simulink model "Motor_ctrl_INST"  (R2025b)
settings: Solver=ode15s  StartTime=0.0  StopTime=1  FixedStep=Ts/10  MaxStep=Tstep  RelTol=1e-3  AbsTol=1e-3  EnableMultiTasking=on
InitFcn:
  | if ~exist('flagwp')
  |     tic
  |     init_sim
  | end
  | mex Motor_ctrl.c User_functions/Src/*.c
StopFcn:
  | if ~exist('flagwp')
  |   elapsed_time=toc
  | end
values from neighbouring files (symbols this model uses):
  accel = 5000    [init_sim.m]
  Bm = 0    [init_sim.m]
  Clarke_inv = [1 0;-0.5 sqrt(3)/2;-0.5 -sqrt(3)/2]    [init_sim.m]
  Ctrl_strategy = 1    [init_sim.m]
  Ctrl_type = 3    [init_sim.m]
  dem = 1    [init_sim.m]
  dT = motorModel.SyreDrive.Converter.dT * 1e-6    [init_sim.m]
  expC = motorModel.IronPMLossMap_dq.expC    [init_sim.m]
  expH = motorModel.IronPMLossMap_dq.expH    [init_sim.m]
  expPM = motorModel.IronPMLossMap_dq.expPM    [init_sim.m]
  Fd0 = interp2(motorModel.FluxMap_dq.Id,motorModel.FluxMap_dq.Iq,motorModel.FluxMap_dq.Fd,0,0)    [init_sim.m]
  Fm = interp2(Idd,Iqq,Fdd,0,0)    [init_sim.m]
  HS_ctrl = 1    [init_sim.m]
  Id_dqt = interpn(motorModel.FluxMapInv_dqt.dataF.Fd,motorModel.FluxMapInv_dqt.dataF.Fq,motorModel.FluxMapInv_dqt.dataF.th,motorModel.FluxMapInv_dqt.dataF.Id,Fd_dqt,Fq_dqt,th_dqt,'cubic')    [init_sim.m]
  Id_fe = motorModel.IronPMLossMap_dq.Id    [init_sim.m]
  InitIntg_d = Fm*cos(th0)    [init_sim.m]
  InitIntg_q = Fm*sin(th0)    [init_sim.m]
  inj_waveform = 1    [init_sim.m]
  Iq_dqt = interpn(motorModel.FluxMapInv_dqt.dataF.Fd,motorModel.FluxMapInv_dqt.dataF.Fq,motorModel.FluxMapInv_dqt.dataF.th,motorModel.FluxMapInv_dqt.dataF.Iq,Fd_dqt,Fq_dqt,th_dqt,'cubic')    [init_sim.m]
  Iq_fe = motorModel.IronPMLossMap_dq.Iq    [init_sim.m]
  IronLoss = 1    [init_sim.m]
  J = motorModel.data.J    [init_sim.m]
  n0 = motorModel.IronPMLossMap_dq.n0    [init_sim.m]
  p = motorModel.data.p    [init_sim.m]
  Pfe_c = motorModel.IronPMLossMap_dq.Pfes_c + motorModel.IronPMLossMap_dq.Pfer_c    [init_sim.m]
  Pfe_h = motorModel.IronPMLossMap_dq.Pfes_h + motorModel.IronPMLossMap_dq.Pfer_h    [init_sim.m]
  Ppm = motorModel.IronPMLossMap_dq.Ppm    [init_sim.m]
  Quad_Maps = 2    [init_sim.m]
  SS_on = 1    [init_sim.m]
  T_dqt = interpn(motorModel.FluxMapInv_dqt.dataF.Fd,motorModel.FluxMapInv_dqt.dataF.Fq,motorModel.FluxMapInv_dqt.dataF.th,motorModel.FluxMapInv_dqt.dataF.T,Fd_dqt,Fq_dqt,th_dqt,'cubic')    [init_sim.m]
  Tf = 0    [init_sim.m]
  th0 = 0    [init_sim.m]
  th_max = max(motorModel.FluxMapInv_dqt.dataF.th,[],'all')    [init_sim.m]
  th_min = min(motorModel.FluxMapInv_dqt.dataF.th,[],'all')    [init_sim.m]
  Ts = 1/motorModel.SyreDrive.Converter.fPWM    [init_sim.m]
  Tv = 0    [init_sim.m]
  VDC = motorModel.data.Vdc    [init_sim.m]
undefined symbols (not defined in the file or in its folder): ACloss, eMotor, fD_pu_norm, fD_vct_max, fD_vct_ref, fQ_pu_norm, fQ_vct_max, fQ_vct_ref, iD_pu_norm, idRef, interpn, iQ_pu_norm, iqRef, J_rot, magnitude, motorModelType, nRef, sigbuilder_block, T0
libraries: nesl_utility x43, fl_lib x41, ee_lib x8, simulink x8, eeTransforms x1
(part 4 of 4)

== system Motor_ctrl_INST/Power block - Inverter + Motor/Noncircuital/FM/Motor Model/Inverse Flux Maps/2D LUT/dq Model/SyR/Fdq -> idq ==
  Fdq : Inport
  1-D Lookup Table : Lookup_n-D  NumberOfTableDimensions=1  BreakpointsForDimension1=fD_vct_ref  Table=fQ_vct_max  InternalRulePriority=Speed  RndMeth=Simplest
  Abs1 : Abs  SaturateOnIntegerOverflow=off
  Abs2 : Abs  SaturateOnIntegerOverflow=off
  Bias : Bias  Bias=-fD_vct_ref(1)  SaturateOnIntegerOverflow=off
  Constant : Constant  Value=fD_vct_ref(end)-fD_vct_ref(1)
  Demux : Demux  Outputs=2
  Divide : Product  Inputs=*/
  Divide1 : Product  Inputs=/*
  Id_pu : Lookup_n-D  BreakpointsForDimension1=fQ_pu_norm(:,1)  BreakpointsForDimension2=fD_pu_norm(1,:)  Table=iD_pu_norm  InternalRulePriority=Speed  RndMeth=Simplest
      settings: InputPortMap=u0,u1
  Iq_pu : Lookup_n-D  BreakpointsForDimension1=fQ_pu_norm(:,1)  BreakpointsForDimension2=fD_pu_norm(1,:)  Table=iQ_pu_norm  InternalRulePriority=Speed  RndMeth=Simplest
      settings: InputPortMap=u0,u1
  Mux : Mux  Inputs=2
  Product1 : Product
  Product2 : Product
  Saturation : Saturate  UpperLimit=fD_vct_ref(end)  LowerLimit=fD_vct_ref(1)
  Saturation Dynamic : simulink/Discontinuities/Saturation Dynamic  OutMin=[]  OutMax=[]  OutDataTypeStr=Inherit: Same as second input  OutDataType=fixdt(1, 16)  OutScaling=2^-10  DoSatur=off
  Sign1 : Signum
  Sign2 : Signum
  Torque calculation : Subsystem
  idq : Outport
  T : Outport  Port=2
  wires:
  1-D Lookup Table/1 -> Divide1/1, Saturation Dynamic/1
  Divide/1 -> Iq_pu/2, Id_pu/2
  Torque calculation/1(Tm) -> T/1
  Abs1/1 -> Saturation Dynamic/3, Saturation Dynamic/2
  Fdq/1 -> Torque calculation/2(Fdq), Demux/1
  Demux/2 -> Sign1/1, Abs1/1
  Iq_pu/1 -> Product1/1
  Abs2/1 -> Saturation/1
  Saturation/1 -> Bias/1, 1-D Lookup Table/1
  Divide1/1 -> Id_pu/1, Iq_pu/1
  Id_pu/1 -> Product2/2
  Bias/1 -> Divide/1
  Saturation Dynamic/1 -> Divide1/2
  Constant/1 -> Divide/2
  Sign1/1 -> Product1/2
  Mux/1 -> Torque calculation/1(Idq), idq/1
  Demux/1 -> Abs2/1, Sign2/1
  Product2/1 -> Mux/1  "iq_pu"
  Sign2/1 -> Product2/1
  Product1/1 -> Mux/2  "iq_pu"

== system Motor_ctrl_INST/Power block - Inverter + Motor/Noncircuital/FM/Motor Model/Inverse Flux Maps/2D LUT/dq Model/SyR/Subsystem1 ==
  theta_r : Inport
  Gain1 : Gain  Gain=p
  Mux3 : Mux  Inputs=2
  Scope : Scope
  Scope1 : Scope
  Sin : Trigonometry
  Sin1 : Trigonometry  Operator=cos
  SinCos : Outport
  wires:
  Sin1/1 -> Mux3/2
  Sin/1 -> Mux3/1
  Mux3/1 -> Scope/1, SinCos/1
  Gain1/1 -> Scope1/1, Sin/1, Sin1/1
  theta_r/1 -> Gain1/1

== system Motor_ctrl_INST/Power block - Inverter + Motor/Noncircuital/FM/Motor Model/Inverse Flux Maps/2D LUT/dq Model/SyR/ab->dq1 ==
  X_ab : Inport
  sin,cos : Inport  Port=2
  Demux : Demux  Outputs=2
  Demux1 : Demux  Outputs=2
  Mux : Mux  Commented=on  Inputs=2
  Mux1 : Mux  Commented=on  Inputs=2
  Mux2 : Mux  Inputs=2
  Product{,1..3} (4 alike) : Product
  Subtract : Sum
  Subtract1 : Sum  Inputs=-+
  X_d : Fcn  Commented=on  Expr=u(1)*u(4) + u(2)*u(3)
  X_q : Fcn  Commented=on  Expr=- u(1)*u(3) + u(2)*u(4)
  X_dq : Outport  InitialOutput=0
  wires:
  X_q/1 -> Mux1/2
  X_d/1 -> Mux1/1
  Mux/1 -> X_q/1, X_d/1
  Demux1/2 -> Product1/2, Product/2
  Demux/2 -> Product1/1, Product2/1
  Demux1/1 -> Product3/2, Product2/2
  Product/1 -> Subtract/1
  Product2/1 -> Subtract/2
  Demux/1 -> Product3/1, Product/1
  Product3/1 -> Subtract1/1
  Product1/1 -> Subtract1/2
  Subtract/1 -> Mux2/1
  Subtract1/1 -> Mux2/2
  X_ab/1 -> Demux/1
  sin,cos/1 -> Demux1/1
  Mux2/1 -> X_dq/1

== system Motor_ctrl_INST/Power block - Inverter + Motor/Noncircuital/FM/Motor Model/Inverse Flux Maps/2D LUT/dq Model/SyR/abc->ab0 ==
  eabc : Inport
  Demux1 : Demux  Outputs=3
  Gain : Gain  Gain=0.5
  Gain1 : Gain  Gain=2/3
  Gain2 : Gain  Gain=1/sqrt(3)
  Gain3 : Gain  Gain=1/3
  Mux1 : Mux  Inputs=3
  Subtract : Sum  Inputs=+-
  Subtract1 : Sum
  Subtract2 : Sum  Inputs=+-
  Subtract3 : Sum  Inputs=+++
  eab0 : Outport
  wires:
  Subtract1/1 -> Gain/1
  Subtract/1 -> Gain1/1
  Demux1/2 -> Subtract3/2, Subtract2/1, Subtract1/1
  Subtract2/1 -> Gain2/1
  Subtract3/1 -> Gain3/1
  Gain1/1 -> Mux1/1
  Demux1/1 -> Subtract/1, Subtract3/1
  Gain3/1 -> Mux1/3
  Gain2/1 -> Mux1/2
  Gain/1 -> Subtract/2
  Mux1/1 -> eab0/1
  Demux1/3 -> Subtract3/3, Subtract2/2, Subtract1/2
  eabc/1 -> Demux1/1

== system Motor_ctrl_INST/Power block - Inverter + Motor/Noncircuital/FM/Motor Model/Inverse Flux Maps/3D LUTs/Variant Subsystem/IPM/Fdq -> idq ==
  Fdq : Inport
  th_e : Inport  Port=2
  Abs4 : Abs  SaturateOnIntegerOverflow=off
  Demux1 : Demux  Outputs=2
  Interpolation Using Prelookup : Interpolation_n-D  NumberOfTableDimensions=3  Table=T_dqt  LookupTableObject=T_th  RequireIndexFractionAsBus=on  InternalRulePriority=Speed
      settings: InputPortMap=u0,u1,u2
  Interpolation Using Prelookup3 : Interpolation_n-D  NumberOfTableDimensions=3  Table=Id_dqt  RequireIndexFractionAsBus=on  InternalRulePriority=Speed
      settings: InputPortMap=u0,u1,u2
  Interpolation Using Prelookup4 : Interpolation_n-D  NumberOfTableDimensions=3  Table=Iq_dqt  RequireIndexFractionAsBus=on  InternalRulePriority=Speed
      settings: InputPortMap=u0,u1,u2
  MATLAB Function2 : MATLAB Function  TreatAsAtomicUnit=on
  Mux1 : Mux  Inputs=2
  Prelookup1 : PreLookup  BreakpointsData=Fd_v  OutputSelection=Index and fraction as bus  BeginIndexSearchUsingPreviousIndexResult=on  ExtrapMethod=Linear
  Prelookup2 : PreLookup  BreakpointsData=Fq_v  OutputSelection=Index and fraction as bus  BeginIndexSearchUsingPreviousIndexResult=on  ExtrapMethod=Linear
  Prelookup6 : PreLookup  BreakpointsData=th_v  OutputSelection=Index and fraction as bus  ExtrapMethod=Linear
  Product1 : Product
  Product5 : Product
  Sign3 : Signum
  th_lim : Saturate  UpperLimit=th_max  LowerLimit=th_min  ZeroCross=off
  idq : Outport
  T : Outport  Port=2
  wires:
  [bus_q] -> Interpolation Using Prelookup4/1
  Product5/1 -> Mux1/2
  Demux1/1 -> Prelookup1/1  "fd"
  [bus_d] -> Interpolation Using Prelookup3/2
  Demux1/2 -> Sign3/1, Abs4/1  "fq"
  Sign3/1 -> Product5/2, Product1/1
  Interpolation Using Prelookup4/1 -> Product5/1
  Interpolation Using Prelookup3/1 -> Mux1/1
  Prelookup2/1 -> [bus_q]
  Abs4/1 -> Prelookup2/1  "fd"
  Mux1/1 -> idq/1
  Prelookup1/1 -> [bus_d]
  [bus_d] -> Interpolation Using Prelookup4/2
  [bus_q] -> Interpolation Using Prelookup3/1
  Fdq/1 -> Demux1/1
  [bus_q] -> Interpolation Using Prelookup/1
  [bus_d] -> Interpolation Using Prelookup/2
  Interpolation Using Prelookup/1 -> Product1/2
  Product1/1 -> T/1
  th_lim/1 -> Prelookup6/1
  MATLAB Function2/1(th_deg) -> th_lim/1
  th_e/1 -> MATLAB Function2/1(th_rad)
  Prelookup6/1 -> [bus_th]
  [bus_th] -> Interpolation Using Prelookup/3
  [bus_th] -> Interpolation Using Prelookup4/3
  [bus_th] -> Interpolation Using Prelookup3/3

== system Motor_ctrl_INST/Power block - Inverter + Motor/Noncircuital/FM/Motor Model/Inverse Flux Maps/3D LUTs/Variant Subsystem/IPM/Subsystem1 ==
  theta_r : Inport
  Gain1 : Gain  Gain=p
  Mux3 : Mux  Inputs=2
  Scope : Scope
  Scope1 : Scope
  Sin : Trigonometry
  Sin1 : Trigonometry  Operator=cos
  SinCos : Outport
  wires:
  Sin1/1 -> Mux3/2
  Sin/1 -> Mux3/1
  Mux3/1 -> Scope/1, SinCos/1
  Gain1/1 -> Scope1/1, Sin/1, Sin1/1
  theta_r/1 -> Gain1/1

== system Motor_ctrl_INST/Power block - Inverter + Motor/Noncircuital/FM/Motor Model/Inverse Flux Maps/3D LUTs/Variant Subsystem/IPM/ab->dq1 ==
  X_ab : Inport
  sin,cos : Inport  Port=2
  Demux : Demux  Outputs=2
  Demux1 : Demux  Outputs=2
  Mux : Mux  Commented=on  Inputs=2
  Mux1 : Mux  Commented=on  Inputs=2
  Mux2 : Mux  Inputs=2
  Product{,1..3} (4 alike) : Product
  Subtract : Sum
  Subtract1 : Sum  Inputs=-+
  X_d : Fcn  Commented=on  Expr=u(1)*u(4) + u(2)*u(3)
  X_q : Fcn  Commented=on  Expr=- u(1)*u(3) + u(2)*u(4)
  X_dq : Outport  InitialOutput=0
  wires:
  X_q/1 -> Mux1/2
  X_d/1 -> Mux1/1
  Mux/1 -> X_q/1, X_d/1
  Demux1/2 -> Product1/2, Product/2
  Demux/2 -> Product1/1, Product2/1
  Demux1/1 -> Product3/2, Product2/2
  Product/1 -> Subtract/1
  Product2/1 -> Subtract/2
  Demux/1 -> Product3/1, Product/1
  Product3/1 -> Subtract1/1
  Product1/1 -> Subtract1/2
  Subtract/1 -> Mux2/1
  Subtract1/1 -> Mux2/2
  X_ab/1 -> Demux/1
  sin,cos/1 -> Demux1/1
  Mux2/1 -> X_dq/1

== system Motor_ctrl_INST/Power block - Inverter + Motor/Noncircuital/FM/Motor Model/Inverse Flux Maps/3D LUTs/Variant Subsystem/IPM/abc->ab0 ==
  eabc : Inport
  Demux1 : Demux  Outputs=3
  Gain : Gain  Gain=0.5
  Gain1 : Gain  Gain=2/3
  Gain2 : Gain  Gain=1/sqrt(3)
  Gain3 : Gain  Gain=1/3
  Mux1 : Mux  Inputs=3
  Subtract : Sum  Inputs=+-
  Subtract1 : Sum
  Subtract2 : Sum  Inputs=+-
  Subtract3 : Sum  Inputs=+++
  eab0 : Outport
  wires:
  Subtract1/1 -> Gain/1
  Subtract/1 -> Gain1/1
  Demux1/2 -> Subtract3/2, Subtract2/1, Subtract1/1
  Subtract2/1 -> Gain2/1
  Subtract3/1 -> Gain3/1
  Gain1/1 -> Mux1/1
  Demux1/1 -> Subtract/1, Subtract3/1
  Gain3/1 -> Mux1/3
  Gain2/1 -> Mux1/2
  Gain/1 -> Subtract/2
  Mux1/1 -> eab0/1
  Demux1/3 -> Subtract3/3, Subtract2/2, Subtract1/2
  eabc/1 -> Demux1/1

== system Motor_ctrl_INST/Power block - Inverter + Motor/Noncircuital/FM/Motor Model/Inverse Flux Maps/3D LUTs/Variant Subsystem/PM-SyR/Fdq -> idq ==
  Fdq : Inport
  theta_elt : Inport  Port=2
  Abs3 : Abs  SaturateOnIntegerOverflow=off
  Demux1 : Demux  Outputs=2
  Interpolation Using Prelookup : Interpolation_n-D  NumberOfTableDimensions=3  Table=T_dqt  LookupTableObject=T_th  RequireIndexFractionAsBus=on  InternalRulePriority=Speed
      settings: InputPortMap=u0,u1,u2
  Interpolation Using Prelookup3 : Interpolation_n-D  NumberOfTableDimensions=3  Table=Id_dqt  RequireIndexFractionAsBus=on  InternalRulePriority=Speed
      settings: InputPortMap=u0,u1,u2
  Interpolation Using Prelookup4 : Interpolation_n-D  NumberOfTableDimensions=3  Table=Iq_dqt  RequireIndexFractionAsBus=on  InternalRulePriority=Speed
      settings: InputPortMap=u0,u1,u2
  MATLAB Function2 : MATLAB Function  TreatAsAtomicUnit=on
  Mux1 : Mux  Inputs=2
  Prelookup1 : PreLookup  BreakpointsData=Fd_v  OutputSelection=Index and fraction as bus  ExtrapMethod=Linear
  Prelookup2 : PreLookup  BreakpointsData=Fq_v  OutputSelection=Index and fraction as bus  ExtrapMethod=Linear
  Prelookup6 : PreLookup  BreakpointsData=th_v  OutputSelection=Index and fraction as bus  ExtrapMethod=Linear
  Product : Product
  Product6 : Product
  Sign2 : Signum
  th_lim : Saturate  UpperLimit=th_max  LowerLimit=th_min  ZeroCross=off
  idq : Outport
  T : Outport  Port=2
  wires:
  Sign2/1 -> Product6/1, Product/1
  [bus_d] -> Interpolation Using Prelookup/2
  [bus_th] -> Interpolation Using Prelookup/3
  Interpolation Using Prelookup4/1 -> Mux1/2
  theta_elt/1 -> MATLAB Function2/1(th_rad)
  Mux1/1 -> idq/1
  Fdq/1 -> Demux1/1
  Prelookup6/1 -> [bus_th]
  Prelookup2/1 -> [bus_q]
  Abs3/1 -> Prelookup1/1  "fd"
  Product6/1 -> T/1
  [bus_d] -> Interpolation Using Prelookup3/2
  [bus_th] -> Interpolation Using Prelookup4/3
  [bus_q] -> Interpolation Using Prelookup/1
  [bus_q] -> Interpolation Using Prelookup4/1
  Interpolation Using Prelookup3/1 -> Product/2
  MATLAB Function2/1(th_deg) -> th_lim/1
  Product/1 -> Mux1/1
  [bus_th] -> Interpolation Using Prelookup3/3
  Demux1/2 -> Prelookup2/1  "fq"
  [bus_q] -> Interpolation Using Prelookup3/1
  [bus_d] -> Interpolation Using Prelookup4/2
  th_lim/1 -> Prelookup6/1
  Interpolation Using Prelookup/1 -> Product6/2
  Demux1/1 -> Sign2/1, Abs3/1  "fd"
  Prelookup1/1 -> [bus_d]
  ? -> ?

== system Motor_ctrl_INST/Power block - Inverter + Motor/Noncircuital/FM/Motor Model/Inverse Flux Maps/3D LUTs/Variant Subsystem/PM-SyR/Subsystem1 ==
  theta_r : Inport
  Gain1 : Gain  Gain=p
  Mux3 : Mux  Inputs=2
  Scope : Scope
  Scope1 : Scope
  Sin : Trigonometry
  Sin1 : Trigonometry  Operator=cos
  SinCos : Outport
  wires:
  Sin1/1 -> Mux3/2
  Sin/1 -> Mux3/1
  Mux3/1 -> Scope/1, SinCos/1
  Gain1/1 -> Scope1/1, Sin/1, Sin1/1
  theta_r/1 -> Gain1/1

== system Motor_ctrl_INST/Power block - Inverter + Motor/Noncircuital/FM/Motor Model/Inverse Flux Maps/3D LUTs/Variant Subsystem/PM-SyR/ab->dq1 ==
  X_ab : Inport
  sin,cos : Inport  Port=2
  Demux : Demux  Outputs=2
  Demux1 : Demux  Outputs=2
  Mux : Mux  Commented=on  Inputs=2
  Mux1 : Mux  Commented=on  Inputs=2
  Mux2 : Mux  Inputs=2
  Product{,1..3} (4 alike) : Product
  Subtract : Sum
  Subtract1 : Sum  Inputs=-+
  X_d : Fcn  Commented=on  Expr=u(1)*u(4) + u(2)*u(3)
  X_q : Fcn  Commented=on  Expr=- u(1)*u(3) + u(2)*u(4)
  X_dq : Outport  InitialOutput=0
  wires:
  X_q/1 -> Mux1/2
  X_d/1 -> Mux1/1
  Mux/1 -> X_q/1, X_d/1
  Demux1/2 -> Product1/2, Product/2
  Demux/2 -> Product1/1, Product2/1
  Demux1/1 -> Product3/2, Product2/2
  Product/1 -> Subtract/1
  Product2/1 -> Subtract/2
  Demux/1 -> Product3/1, Product/1
  Product3/1 -> Subtract1/1
  Product1/1 -> Subtract1/2
  Subtract/1 -> Mux2/1
  Subtract1/1 -> Mux2/2
  X_ab/1 -> Demux/1
  sin,cos/1 -> Demux1/1
  Mux2/1 -> X_dq/1

== system Motor_ctrl_INST/Power block - Inverter + Motor/Noncircuital/FM/Motor Model/Inverse Flux Maps/3D LUTs/Variant Subsystem/PM-SyR/abc->ab0 ==
  eabc : Inport
  Demux1 : Demux  Outputs=3
  Gain : Gain  Gain=0.5
  Gain1 : Gain  Gain=2/3
  Gain2 : Gain  Gain=1/sqrt(3)
  Gain3 : Gain  Gain=1/3
  Mux1 : Mux  Inputs=3
  Subtract : Sum  Inputs=+-
  Subtract1 : Sum
  Subtract2 : Sum  Inputs=+-
  Subtract3 : Sum  Inputs=+++
  eab0 : Outport
  wires:
  Subtract1/1 -> Gain/1
  Subtract/1 -> Gain1/1
  Demux1/2 -> Subtract3/2, Subtract2/1, Subtract1/1
  Subtract2/1 -> Gain2/1
  Subtract3/1 -> Gain3/1
  Gain1/1 -> Mux1/1
  Demux1/1 -> Subtract/1, Subtract3/1
  Gain3/1 -> Mux1/3
  Gain2/1 -> Mux1/2
  Gain/1 -> Subtract/2
  Mux1/1 -> eab0/1
  Demux1/3 -> Subtract3/3, Subtract2/2, Subtract1/2
  eabc/1 -> Demux1/1

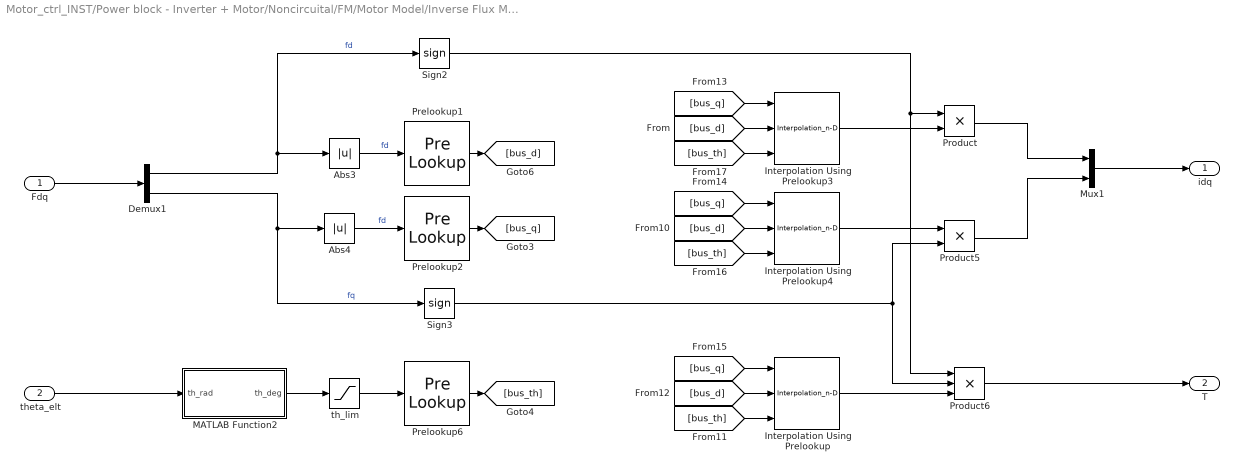
== system Motor_ctrl_INST/Power block - Inverter + Motor/Noncircuital/FM/Motor Model/Inverse Flux Maps/3D LUTs/Variant Subsystem/SyR/Fdq -> idq ==
  Fdq : Inport
  theta_elt : Inport  Port=2
  Abs3 : Abs  SaturateOnIntegerOverflow=off
  Abs4 : Abs  SaturateOnIntegerOverflow=off
  Demux1 : Demux  Outputs=2
  Interpolation Using Prelookup : Interpolation_n-D  NumberOfTableDimensions=3  Table=T_dqt  LookupTableObject=T_th  RequireIndexFractionAsBus=on  InternalRulePriority=Speed
      settings: InputPortMap=u0,u1,u2
  Interpolation Using Prelookup3 : Interpolation_n-D  NumberOfTableDimensions=3  Table=Id_dqt  RequireIndexFractionAsBus=on  InternalRulePriority=Speed
      settings: InputPortMap=u0,u1,u2
  Interpolation Using Prelookup4 : Interpolation_n-D  NumberOfTableDimensions=3  Table=Iq_dqt  RequireIndexFractionAsBus=on  InternalRulePriority=Speed
      settings: InputPortMap=u0,u1,u2
  MATLAB Function2 : MATLAB Function  TreatAsAtomicUnit=on
  Mux1 : Mux  Inputs=2
  Prelookup1 : PreLookup  BreakpointsData=Fd_v  OutputSelection=Index and fraction as bus  ExtrapMethod=Linear
  Prelookup2 : PreLookup  BreakpointsData=Fq_v  OutputSelection=Index and fraction as bus  ExtrapMethod=Linear
  Prelookup6 : PreLookup  BreakpointsData=th_v  OutputSelection=Index and fraction as bus  ExtrapMethod=Linear
  Product : Product
  Product5 : Product
  Product6 : Product  Inputs=3
  Sign2 : Signum
  Sign3 : Signum
  th_lim : Saturate  UpperLimit=th_max  LowerLimit=th_min  ZeroCross=off
  idq : Outport
  T : Outport  Port=2
  wires:
  th_lim/1 -> Prelookup6/1
  Product6/1 -> T/1
  [bus_th] -> Interpolation Using Prelookup/3
  MATLAB Function2/1(th_deg) -> th_lim/1
  Demux1/2 -> Sign3/1, Abs4/1  "fq"
  [bus_q] -> Interpolation Using Prelookup3/1
  Prelookup6/1 -> [bus_th]
  Demux1/1 -> Sign2/1, Abs3/1  "fd"
  theta_elt/1 -> MATLAB Function2/1(th_rad)
  Sign2/1 -> Product6/1, Product/1
  Interpolation Using Prelookup/1 -> Product6/3
  Prelookup1/1 -> [bus_d]
  Abs3/1 -> Prelookup1/1  "fd"
  Fdq/1 -> Demux1/1
  Prelookup2/1 -> [bus_q]
  Interpolation Using Prelookup3/1 -> Product/2
  Abs4/1 -> Prelookup2/1  "fd"
  [bus_d] -> Interpolation Using Prelookup4/2
  Interpolation Using Prelookup4/1 -> Product5/1
  Product/1 -> Mux1/1
  [bus_d] -> Interpolation Using Prelookup/2
  [bus_d] -> Interpolation Using Prelookup3/2
  [bus_q] -> Interpolation Using Prelookup/1
  Sign3/1 -> Product6/2, Product5/2
  [bus_q] -> Interpolation Using Prelookup4/1
  Mux1/1 -> idq/1
  Product5/1 -> Mux1/2
  [bus_th] -> Interpolation Using Prelookup3/3
  [bus_th] -> Interpolation Using Prelookup4/3

== system Motor_ctrl_INST/Power block - Inverter + Motor/Noncircuital/FM/Motor Model/Inverse Flux Maps/3D LUTs/Variant Subsystem/SyR/Subsystem1 ==
  theta_r : Inport
  Gain1 : Gain  Gain=p
  Mux3 : Mux  Inputs=2
  Scope : Scope
  Scope1 : Scope
  Sin : Trigonometry
  Sin1 : Trigonometry  Operator=cos
  SinCos : Outport
  wires:
  Sin1/1 -> Mux3/2
  Sin/1 -> Mux3/1
  Mux3/1 -> Scope/1, SinCos/1
  Gain1/1 -> Scope1/1, Sin/1, Sin1/1
  theta_r/1 -> Gain1/1

== system Motor_ctrl_INST/Power block - Inverter + Motor/Noncircuital/FM/Motor Model/Inverse Flux Maps/3D LUTs/Variant Subsystem/SyR/ab->dq1 ==
  X_ab : Inport
  sin,cos : Inport  Port=2
  Demux : Demux  Outputs=2
  Demux1 : Demux  Outputs=2
  Mux : Mux  Commented=on  Inputs=2
  Mux1 : Mux  Commented=on  Inputs=2
  Mux2 : Mux  Inputs=2
  Product{,1..3} (4 alike) : Product
  Subtract : Sum
  Subtract1 : Sum  Inputs=-+
  X_d : Fcn  Commented=on  Expr=u(1)*u(4) + u(2)*u(3)
  X_q : Fcn  Commented=on  Expr=- u(1)*u(3) + u(2)*u(4)
  X_dq : Outport  InitialOutput=0
  wires:
  X_q/1 -> Mux1/2
  X_d/1 -> Mux1/1
  Mux/1 -> X_q/1, X_d/1
  Demux1/2 -> Product1/2, Product/2
  Demux/2 -> Product1/1, Product2/1
  Demux1/1 -> Product3/2, Product2/2
  Product/1 -> Subtract/1
  Product2/1 -> Subtract/2
  Demux/1 -> Product3/1, Product/1
  Product3/1 -> Subtract1/1
  Product1/1 -> Subtract1/2
  Subtract/1 -> Mux2/1
  Subtract1/1 -> Mux2/2
  X_ab/1 -> Demux/1
  sin,cos/1 -> Demux1/1
  Mux2/1 -> X_dq/1

== system Motor_ctrl_INST/Power block - Inverter + Motor/Noncircuital/FM/Motor Model/Inverse Flux Maps/3D LUTs/Variant Subsystem/SyR/abc->ab0 ==
  eabc : Inport
  Demux1 : Demux  Outputs=3
  Gain : Gain  Gain=0.5
  Gain1 : Gain  Gain=2/3
  Gain2 : Gain  Gain=1/sqrt(3)
  Gain3 : Gain  Gain=1/3
  Mux1 : Mux  Inputs=3
  Subtract : Sum  Inputs=+-
  Subtract1 : Sum
  Subtract2 : Sum  Inputs=+-
  Subtract3 : Sum  Inputs=+++
  eab0 : Outport
  wires:
  Subtract1/1 -> Gain/1
  Subtract/1 -> Gain1/1
  Demux1/2 -> Subtract3/2, Subtract2/1, Subtract1/1
  Subtract2/1 -> Gain2/1
  Subtract3/1 -> Gain3/1
  Gain1/1 -> Mux1/1
  Demux1/1 -> Subtract/1, Subtract3/1
  Gain3/1 -> Mux1/3
  Gain2/1 -> Mux1/2
  Gain/1 -> Subtract/2
  Mux1/1 -> eab0/1
  Demux1/3 -> Subtract3/3, Subtract2/2, Subtract1/2
  eabc/1 -> Demux1/1

== system Motor_ctrl_INST/Power block - Inverter + Motor/Circuital/Motor model/CCG model/Motor Model/Inverse Flux Maps/2D LUT/dq Model/IPM/Torque calculation ==
  Idq : Inport
  Fdq : Inport  Port=2
  Add : Sum  Inputs=+-
  Demux1 : Demux  Outputs=2
  Demux3 : Demux  Outputs=2
  Gain2 : Gain  Gain=1.5*p
  Product : Product
  Product1 : Product
  Tm : Outport
  wires:
  Demux1/1 -> Product/1
  Product/1 -> Add/1
  Demux3/1 -> Product1/2
  Demux3/2 -> Product/2
  Demux1/2 -> Product1/1
  Product1/1 -> Add/2
  Fdq/1 -> Demux1/1
  Add/1 -> Gain2/1
  Idq/1 -> Demux3/1
  Gain2/1 -> Tm/1

== system Motor_ctrl_INST/Power block - Inverter + Motor/Circuital/Motor model/CCG model/Motor Model/Inverse Flux Maps/2D LUT/dq Model/PM-SyR/Torque calculation ==
  Idq : Inport
  Fdq : Inport  Port=2
  Add : Sum  Inputs=+-
  Demux1 : Demux  Outputs=2
  Demux3 : Demux  Outputs=2
  Gain2 : Gain  Gain=1.5*p
  Product : Product
  Product1 : Product
  Tm : Outport
  wires:
  Demux1/1 -> Product/1
  Product/1 -> Add/1
  Demux3/1 -> Product1/2
  Demux3/2 -> Product/2
  Demux1/2 -> Product1/1
  Product1/1 -> Add/2
  Fdq/1 -> Demux1/1
  Add/1 -> Gain2/1
  Idq/1 -> Demux3/1
  Gain2/1 -> Tm/1

== system Motor_ctrl_INST/Power block - Inverter + Motor/Circuital/Motor model/CCG model/Motor Model/Inverse Flux Maps/2D LUT/dq Model/SyR/Torque calculation ==
  Idq : Inport
  Fdq : Inport  Port=2
  Add : Sum  Inputs=+-
  Demux1 : Demux  Outputs=2
  Demux3 : Demux  Outputs=2
  Gain2 : Gain  Gain=1.5*p
  Product : Product
  Product1 : Product
  Tm : Outport
  wires:
  Demux1/1 -> Product/1
  Product/1 -> Add/1
  Demux3/1 -> Product1/2
  Demux3/2 -> Product/2
  Demux1/2 -> Product1/1
  Product1/1 -> Add/2
  Fdq/1 -> Demux1/1
  Add/1 -> Gain2/1
  Idq/1 -> Demux3/1
  Gain2/1 -> Tm/1

== system Motor_ctrl_INST/Power block - Inverter + Motor/Noncircuital/FM/Motor Model/Inverse Flux Maps/2D LUT/dq Model/IPM/Fdq -> idq/Torque calculation ==
  Idq : Inport
  Fdq : Inport  Port=2
  Add : Sum  Inputs=+-
  Demux1 : Demux  Outputs=2
  Demux3 : Demux  Outputs=2
  Gain2 : Gain  Gain=1.5*p
  Product : Product
  Product1 : Product
  Tm : Outport
  wires:
  Demux1/1 -> Product/1
  Product/1 -> Add/1
  Demux3/1 -> Product1/2
  Demux3/2 -> Product/2
  Demux1/2 -> Product1/1
  Product1/1 -> Add/2
  Fdq/1 -> Demux1/1
  Add/1 -> Gain2/1
  Idq/1 -> Demux3/1
  Gain2/1 -> Tm/1

== system Motor_ctrl_INST/Power block - Inverter + Motor/Noncircuital/FM/Motor Model/Inverse Flux Maps/2D LUT/dq Model/PM-SyR/Fdq -> idq/Torque calculation ==
  Idq : Inport
  Fdq : Inport  Port=2
  Add : Sum  Inputs=+-
  Demux1 : Demux  Outputs=2
  Demux3 : Demux  Outputs=2
  Gain2 : Gain  Gain=1.5*p
  Product : Product
  Product1 : Product
  Tm : Outport
  wires:
  Demux1/1 -> Product/1
  Product/1 -> Add/1
  Demux3/1 -> Product1/2
  Demux3/2 -> Product/2
  Demux1/2 -> Product1/1
  Product1/1 -> Add/2
  Fdq/1 -> Demux1/1
  Add/1 -> Gain2/1
  Idq/1 -> Demux3/1
  Gain2/1 -> Tm/1

== system Motor_ctrl_INST/Power block - Inverter + Motor/Noncircuital/FM/Motor Model/Inverse Flux Maps/2D LUT/dq Model/SyR/Fdq -> idq/Torque calculation ==
  Idq : Inport
  Fdq : Inport  Port=2
  Add : Sum  Inputs=+-
  Demux1 : Demux  Outputs=2
  Demux3 : Demux  Outputs=2
  Gain2 : Gain  Gain=1.5*p
  Product : Product
  Product1 : Product
  Tm : Outport
  wires:
  Demux1/1 -> Product/1
  Product/1 -> Add/1
  Demux3/1 -> Product1/2
  Demux3/2 -> Product/2
  Demux1/2 -> Product1/1
  Product1/1 -> Add/2
  Fdq/1 -> Demux1/1
  Add/1 -> Gain2/1
  Idq/1 -> Demux3/1
  Gain2/1 -> Tm/1

== matlab function Motor_ctrl_INST/Power block - Inverter + Motor/Circuital/Motor model/CCG model/Motor Model/Inverse Flux Maps/3D LUTs/Variant Subsystem/IPM/MATLAB Function2 ==
  data: th_rad input; th_deg output
function th_deg = fcn(th_rad)

th_deg=th_rad*180/pi;

while th_deg>360
    th_deg=th_deg-360;
end

while th_deg<0
    th_deg=th_deg+360;
end

== matlab function Motor_ctrl_INST/Power block - Inverter + Motor/Circuital/Motor model/CCG model/Motor Model/Inverse Flux Maps/3D LUTs/Variant Subsystem/PM-SyR/MATLAB Function2 ==
  data: th_rad input; th_deg output
function th_deg = fcn(th_rad)

th_deg=th_rad*180/pi;

while th_deg>360
    th_deg=th_deg-360;
end

while th_deg<0
    th_deg=th_deg+360;
end

== matlab function Motor_ctrl_INST/Power block - Inverter + Motor/Circuital/Motor model/CCG model/Motor Model/Inverse Flux Maps/3D LUTs/Variant Subsystem/SyR/MATLAB Function2 ==
  data: th_rad input; th_deg output
function th_deg = fcn(th_rad)

th_deg=th_rad*180/pi;

while th_deg>360
    th_deg=th_deg-360;
end

while th_deg<0
    th_deg=th_deg+360;
end

== matlab function Motor_ctrl_INST/Power block - Inverter + Motor/Circuital/Motor model/CCG model/Motor Model/Iron Losses Maps/Iron Losses/Iron loss Maps/MATLAB Function1 ==
  data: P input; Id_fe output; Fdq input; n input; p input; Iq_fe output
function [Id_fe,Iq_fe] = fcn(P,Fdq,n,p)

Id_fe = 0;
Iq_fe = 0; 

if(n>0)
    tmp1 = (n*pi*p)/30;
    tmp2 = Fdq(1)*Fdq(1)+Fdq(2)*Fdq(2);
    tmp3 = tmp1*tmp2;
    Id_fe = (P/tmp3)*(-Fdq(2));
    Iq_fe = (P/tmp3)*(Fdq(1));

   
end    

end

== matlab function Motor_ctrl_INST/Power block - Inverter + Motor/Circuital/Motor model/CCG model/Motor Model/Iron Losses Maps/Iron Losses/Iron loss Maps/Stator Voltage Eqaution1 ==
  data: idq_m input; Quad_Maps input; idq_out output
function idq_out = fcn(idq_m, Quad_Maps)

idq_out = [0; 0];

switch(Quad_Maps)
    case 0 %SyR
        idq_out(1) = abs(idq_m(1));
        idq_out(2) = abs(idq_m(2));
    case 1  %PM-SyR
        idq_out(1) = abs(idq_m(1));
        idq_out(2) = idq_m(2);
    case 2  %PM  
        idq_out(1) = idq_m(1);
        idq_out(2) = abs(idq_m(2));
end

end

== matlab function Motor_ctrl_INST/Power block - Inverter + Motor/Noncircuital/FM/Motor Model/Inverse Flux Maps/3D LUTs/Variant Subsystem/IPM/Fdq -> idq/MATLAB Function2 ==
  data: th_rad input; th_deg output
function th_deg = fcn(th_rad)

th_deg=th_rad*180/pi;

while th_deg>360
    th_deg=th_deg-360;
end

while th_deg<0
    th_deg=th_deg+360;
end

== matlab function Motor_ctrl_INST/Power block - Inverter + Motor/Noncircuital/FM/Motor Model/Inverse Flux Maps/3D LUTs/Variant Subsystem/PM-SyR/Fdq -> idq/MATLAB Function2 ==
  data: th_rad input; th_deg output
function th_deg = fcn(th_rad)

th_deg=th_rad*180/pi;

while th_deg>360
    th_deg=th_deg-360;
end

while th_deg<0
    th_deg=th_deg+360;
end

== matlab function Motor_ctrl_INST/Power block - Inverter + Motor/Noncircuital/FM/Motor Model/Inverse Flux Maps/3D LUTs/Variant Subsystem/SyR/Fdq -> idq/MATLAB Function2 ==
  data: th_rad input; th_deg output
function th_deg = fcn(th_rad)

th_deg=th_rad*180/pi;

while th_deg>360
    th_deg=th_deg-360;
end

while th_deg<0
    th_deg=th_deg+360;
end

== matlab function Motor_ctrl_INST/Power block - Inverter + Motor/Noncircuital/FM/Motor Model/Iron Losses Maps/Iron Losses/Iron loss Maps/MATLAB Function1 ==
  data: P input; Id_fe output; Fdq input; n input; p input; Iq_fe output
function [Id_fe,Iq_fe] = fcn(P,Fdq,n,p)

Id_fe = 0;
Iq_fe = 0; 

if(n>0)
    tmp1 = (n*pi*p)/30;
    tmp2 = Fdq(1)*Fdq(1)+Fdq(2)*Fdq(2);
    tmp3 = tmp1*tmp2;
    Id_fe = (P/tmp3)*(-Fdq(2));
    Iq_fe = (P/tmp3)*(Fdq(1));

   
end    

end

== matlab function Motor_ctrl_INST/Power block - Inverter + Motor/Noncircuital/FM/Motor Model/Iron Losses Maps/Iron Losses/Iron loss Maps/Stator Voltage Eqaution1 ==
  data: idq_m input; Quad_Maps input; idq_out output
function idq_out = fcn(idq_m, Quad_Maps)

idq_out = [0; 0];

switch(Quad_Maps)
    case 0 %SyR
        idq_out(1) = abs(idq_m(1));
        idq_out(2) = abs(idq_m(2));
    case 1  %PM-SyR
        idq_out(1) = abs(idq_m(1));
        idq_out(2) = idq_m(2);
    case 2  %PM  
        idq_out(1) = idq_m(1);
        idq_out(2) = abs(idq_m(2));
end

end
